simulink model "ScriptDemo"  (R2022b)
settings: configuration reference "TmVcThermal_Configuration_sub" (kept outside this file)
undefined symbols (not defined in the file or in its folder): aaaa, bbbb, cTmComprCtrl_D_u8HvacFlowTable_db, cTmComprCtrl_D_u8HvacFlowTable_sw, cTmComprCtrl_n_i16ChillCmpIMax, cTmComprCtrl_n_i16ChillCmpIMin, cTmComprCtrl_n_i16ChillCmpIMin666, cTmComprCtrl_n_i16ChillCmpPMax, cTmComprCtrl_n_i16ChillCmpPMin, cTmComprCtrl_n_i16CmpChillCoolRpmKiMax, cTmComprCtrl_n_i16CmpChillCoolRpmKiMin, cTmComprCtrl_n_i16CmpChillCoolRpmKpMax, cTmComprCtrl_n_i16CmpChillCoolRpmKpMin, cTmComprCtrl_n_i16CmpCoolRpmKiMax, cTmComprCtrl_n_i16CmpCoolRpmKiMin, cTmComprCtrl_n_i16CmpCoolRpmKpMax, cTmComprCtrl_n_i16CmpCoolRpmKpMin, cTmComprCtrl_n_i16SM4CmpHeatKiMax, cTmComprCtrl_n_i16SM4CmpHeatKiMin, cTmComprCtrl_n_i16SM4CmpHeatKpMax, cTmComprCtrl_n_i16SM4CmpHeatKpMin, cTmComprCtrl_n_i16SM5CmpHeatKiMax, cTmComprCtrl_n_i16SM5CmpHeatKiMin, cTmComprCtrl_n_i16SM5CmpHeatKpMax, cTmComprCtrl_n_i16SM5CmpHeatKpMin, cTmComprCtrl_n_i16SM6CmpHeatKiMax, cTmComprCtrl_n_i16SM6CmpHeatKiMin, cTmComprCtrl_n_i16SM6CmpHeatKpMax, cTmComprCtrl_n_i16SM6CmpHeatKpMin, cTmComprCtrl_n_u16CmpMaxSpdFanFltLimt, cTmComprCtrl_n_u16CmpMaxSpdLoSidePFltLimt, cTmComprCtrl_n_u16CmpMaxSpdSensorFltLimt, cTmComprCtrl_n_u16CompMinRpm, cTmComprCtrl_n_u16CompRpmIncThres, cTmComprCtrl_t_u16BattCooltFFPeriod, cTmComprCtrl_t_u16BattCooltPIPeriod, cTmComprCtrl_t_u16CmpCoolFFPeriod, cTmComprCtrl_t_u16CmpCoolPIPeriod, cTmComprCtrl_t_u16CoolCmpChillFFPeriod, cTmComprCtrl_t_u16CoolCmpChillPIPeriod, cTmComprCtrl_t_u16SM4CmpHeatFFPeriod, cTmComprCtrl_t_u16SM4CmpHeatPIPeriod, cTmComprCtrl_t_u16SM5CmpHeatFFPeriod, cTmComprCtrl_t_u16SM5CmpHeatPIPeriod, cTmComprCtrl_t_u16SM6CmpHeatFFPeriod, cTmComprCtrl_t_u16SM6CmpHeatPIPeriod, cTmComprCtrl_Te_EvapClearInteg, cTmComprCtrl_Te_i16HpReqTempSaturoffset, cTmComprCtrl_Te_i16SatLpReplaceDiff, cTmComprCtrl_Te_i16SM3BatDiffStartEvapDecOffset, cTmComprCtrl_Te_i16SM3EvapLo, cTmComprCtrl_Te_i16SM3TBatDiffEntEvapDecOffset, cTmComprCtrl_Te_i16SM3TBatDiffEntEvapDecOffsetQuit, cTmComprCtrl_Te_s32ErrCmpChillPIContinueCoolH, cTmComprCtrl_Te_s32ErrCmpChillPIContinueCoolL, cTmComprCtrl_Te_s32ErrCmpPIContinueChillH, cTmComprCtrl_Te_s32ErrCmpPIContinueChillL, cTmComprCtrl_Te_s32ErrCmpPIContinueCoolH, cTmComprCtrl_Te_s32ErrCmpPIContinueCoolL, cTmComprCtrl_Te_s32ErrCmpPIContinueHeatH ... (+398)
libraries: simulink x846, PCMULib x711, simulink_need_slupdate x4
(part 18 of 49)

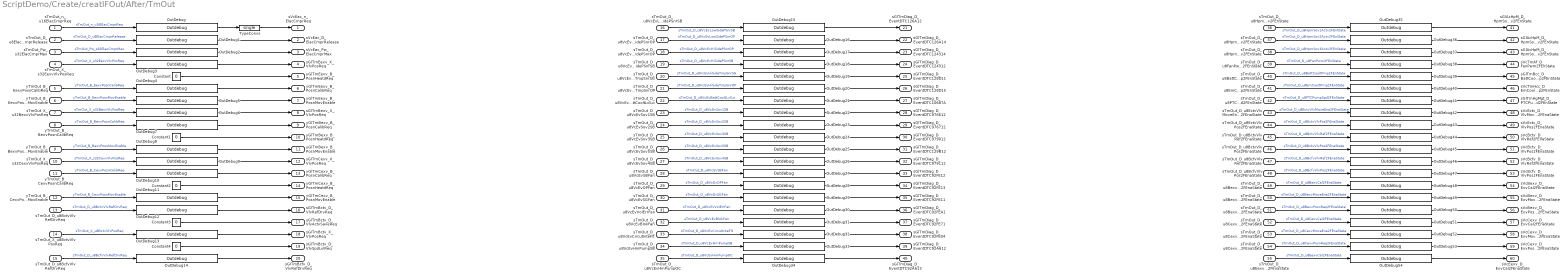
== system ScriptDemo/Create/creatIFOut/After/TmOut ==
  sTmOut_n_u16ElacCmprReq : Inport  OutDataTypeStr=uint16
  sTmOut_D_u8ElacCmprRelease : Inport  Port=2  OutDataTypeStr=uint8
  sTmOut_Pw_s32ElacCmprMax : Inport  Port=3  OutDataTypeStr=single
  sTmOut_X_s32EexvVlvPosReq : Inport  Port=4  OutDataTypeStr=single
  yTmOut_B_EexvPosnCalibReq : Inport  Port=5  OutDataTypeStr=boolean
  yTmOut_B_EexvPosnMovEnable : Inport  Port=6  OutDataTypeStr=boolean
  sTmOut_X_s32BexvVlvPosReq : Inport  Port=7  OutDataTypeStr=single
  yTmOut_B_BexvPosnCalibReq : Inport  Port=8  OutDataTypeStr=boolean
  yTmOut_B_BexvPosnMovEnable : Inport  Port=9  OutDataTypeStr=boolean
  sTmOut_X_s32CexvVlvPosReq : Inport  Port=10  OutDataTypeStr=single
  yTmOut_B_CexvPosnCalibReq : Inport  Port=11  OutDataTypeStr=boolean
  yTmOut_B_CexvPosnMovEnable : Inport  Port=12  OutDataTypeStr=boolean
  sTmOut_D_u8BctvVlvRefDrvReq : Inport  Port=13  OutDataTypeStr=uint8
  sTmOut_X_u8BctvVlvPosReq : Inport  Port=14  OutDataTypeStr=uint8
  sTmOut_D_u8BcfvVlvRefDrvReq : Inport  Port=15  OutDataTypeStr=uint8
  sTmOut_D_u8VcEvLowSidePSnrSB : Inport  Port=16  OutDataTypeStr=uint8
  sTmOut_D_u8VcEvLowSidePSnrOP : Inport  Port=17  OutDataTypeStr=uint8
  sTmOut_D_u8VcEvHiSidePSnrOP : Inport  Port=18  OutDataTypeStr=uint8
  sTmOut_D_u8VcEvHiSidePSnrSB : Inport  Port=19  OutDataTypeStr=uint8
  sTmOut_D_u8VcEvHiSideTmpSnrSG : Inport  Port=20  OutDataTypeStr=uint8
  sTmOut_D_u8VcEvHiSideTmpSnrOP : Inport  Port=21  OutDataTypeStr=uint8
  sTmOut_D_u8VcEvBattCooltLvlLo : Inport  Port=22  OutDataTypeStr=uint8
  sTmOut_D_u8VcEvSov1SB : Inport  Port=23  OutDataTypeStr=uint8
  sTmOut_D_u8VcEvSov2SB : Inport  Port=24  OutDataTypeStr=uint8
  sTmOut_D_u8VcEvSov3SB : Inport  Port=25  OutDataTypeStr=uint8
  sTmOut_D_u8VcEvSov5SB : Inport  Port=26  OutDataTypeStr=uint8
  sTmOut_D_u8VcEvSov4SB : Inport  Port=27  OutDataTypeStr=uint8
  sTmOut_D_u8VcEvSBFan : Inport  Port=28  OutDataTypeStr=uint8
  sTmOut_D_u8VcEvOPFan : Inport  Port=29  OutDataTypeStr=uint8
  sTmOut_D_u8VcEvSGFan : Inport  Port=30  OutDataTypeStr=uint8
  sTmOut_D_u8VcEvVolErrFan : Inport  Port=31  OutDataTypeStr=uint8
  sTmOut_D_u8VcEvBlokFan : Inport  Port=32  OutDataTypeStr=uint8
  sTmOut_D_u8VcEvCircutInteFlt : Inport  Port=33  OutDataTypeStr=uint8
  sTmOut_D_u8VcEvHmPumpSB : Inport  Port=34  OutDataTypeStr=uint8
  sTmOut_D_u8VcEvHmPumpOC : Inport  Port=35  OutDataTypeStr=uint8
  sTmOut_D_u8HpmSov1Actv2FEnState : Inport  Port=36  OutDataTypeStr=uint8
  sTmOut_D_u8HpmSov2Actv2FEnState : Inport  Port=37  OutDataTypeStr=uint8
  sTmOut_D_u8HpmSov3Actv2FEnState : Inport  Port=38  OutDataTypeStr=uint8
  sTmOut_D_u8FanPwm2FEnState : Inport  Port=39  OutDataTypeStr=uint8
  sTmOut_D_u8BattCooltPmp2FEnState : Inport  Port=40  OutDataTypeStr=uint8
  sTmOut_D_u8EmCooltPmp2FEnState : Inport  Port=41  OutDataTypeStr=uint8
  sTmOut_D_u8PTCPumpSpd2FEnState : Inport  Port=42  OutDataTypeStr=uint8
  sTmOut_D_u8EctvVlvMoveEna2FEnaState : Inport  Port=43  OutDataTypeStr=uint8
  sTmOut_D_u8EctvVlvPos2FEnaState : Inport  Port=44  OutDataTypeStr=uint8
  sTmOut_D_u8BctvVlvRef2FEnaState : Inport  Port=45  OutDataTypeStr=uint8
  sTmOut_D_u8BctvVlvPos2FEnaState : Inport  Port=46  OutDataTypeStr=uint8
  sTmOut_D_u8BcfvVlvRef2FEnaState : Inport  Port=47  OutDataTypeStr=uint8
  sTmOut_D_u8BcfvVlvPos2FEnaState : Inport  Port=48  OutDataTypeStr=uint8
  sTmOut_D_u8BexvCal2FEnaState : Inport  Port=49  OutDataTypeStr=uint8
  sTmOut_D_u8BexvMoveEna2FEnaState : Inport  Port=50  OutDataTypeStr=uint8
  sTmOut_D_u8BexvPosnReq2FEnaState : Inport  Port=51  OutDataTypeStr=uint8
  sTmOut_D_u8CexvCal2FEnaState : Inport  Port=52  OutDataTypeStr=uint8
  sTmOut_D_u8CexvMoveEna2FEnaState : Inport  Port=53  OutDataTypeStr=uint8
  sTmOut_D_u8CexvPosnReq2FEnaState : Inport  Port=54  OutDataTypeStr=uint8
  sTmOut_D_u8EexvCal2FEnaState : Inport  Port=55  OutDataTypeStr=uint8
  Constant : Constant  Value=0  OutDataTypeStr=boolean
  Constant1 : Constant  Value=0  OutDataTypeStr=boolean
  Constant2 : Constant  Value=0  OutDataTypeStr=boolean
  Constant3 : Constant  Value=0  OutDataTypeStr=uint8
  Constant4 : Constant  Value=0  OutDataTypeStr=uint8
  OutDebug : PCMULib/Interface/Outdebug  SWI=cTmOut_n_u16ElacCmprReq_sw  DBI=cTmOut_n_u16ElacCmprReq_db
      settings: SourceProductName=PCMULib
  OutDebug1 : PCMULib/Interface/Outdebug  SWI=cTmOut_D_u8ElacCmprRelease_sw  DBI=cTmOut_D_u8ElacCmprRelease_db
      settings: SourceProductName=PCMULib
  OutDebug10 : PCMULib/Interface/Outdebug  SWI=cTmOut_B_CexvPosnCalibReq_sw  DBI=cTmOut_B_CexvPosnCalibReq_db
      settings: SourceProductName=PCMULib
  OutDebug11 : PCMULib/Interface/Outdebug  SWI=cTmOut_B_CexvPosnMovEnable_sw  DBI=cTmOut_B_CexvPosnMovEnable_db
      settings: SourceProductName=PCMULib
  OutDebug12 : PCMULib/Interface/Outdebug  SWI=cTmOut_D_u8BctvVlvRefDrvReq_sw  DBI=cTmOut_D_u8BctvVlvRefDrvReq_db
      settings: SourceProductName=PCMULib
  OutDebug13 : PCMULib/Interface/Outdebug  SWI=cTmOut_X_u8BctvVlvPosReq_sw  DBI=cTmOut_X_u8BctvVlvPosReq_db
      settings: SourceProductName=PCMULib
  OutDebug14 : PCMULib/Interface/Outdebug  SWI=cTmOut_D_u8BcfvVlvRefDrvReq_sw  DBI=cTmOut_D_u8BcfvVlvRefDrvReq_db
      settings: SourceProductName=PCMULib
  OutDebug15 : PCMULib/Interface/Outdebug  SWI=cTmOut_D_u8VcEvLowSidePSnrSB_sw  DBI=cTmOut_D_u8VcEvLowSidePSnrSB_db
      settings: SourceProductName=PCMULib
  OutDebug16 : PCMULib/Interface/Outdebug  SWI=cTmOut_D_u8VcEvLowSidePSnrOP_sw  DBI=cTmOut_D_u8VcEvLowSidePSnrOP_db
      settings: SourceProductName=PCMULib
  OutDebug17 : PCMULib/Interface/Outdebug  SWI=cTmOut_D_u8VcEvHiSidePSnrOP_sw  DBI=cTmOut_D_u8VcEvHiSidePSnrOP_db
      settings: SourceProductName=PCMULib
  OutDebug18 : PCMULib/Interface/Outdebug  SWI=cTmOut_D_u8VcEvHiSidePSnrSB_sw  DBI=cTmOut_D_u8VcEvHiSidePSnrSB_db
      settings: SourceProductName=PCMULib
  OutDebug19 : PCMULib/Interface/Outdebug  SWI=cTmOut_D_u8VcEvHiSideTmpSnrSG_sw  DBI=cTmOut_D_u8VcEvHiSideTmpSnrSG_db
      settings: SourceProductName=PCMULib
  OutDebug2 : PCMULib/Interface/Outdebug  SWI=cTmOut_Pw_s32ElacCmprMax_sw  DBI=cTmOut_Pw_s32ElacCmprMax_db
      settings: SourceProductName=PCMULib
  OutDebug20 : PCMULib/Interface/Outdebug  SWI=cTmOut_D_u8VcEvHiSideTmpSnrOP_sw  DBI=cTmOut_D_u8VcEvHiSideTmpSnrOP_db
      settings: SourceProductName=PCMULib
  OutDebug21 : PCMULib/Interface/Outdebug  SWI=cTmOut_D_u8VcEvBattCooltLvlLo_sw  DBI=cTmOut_D_u8VcEvBattCooltLvlLo_db
      settings: SourceProductName=PCMULib
  OutDebug22 : PCMULib/Interface/Outdebug  SWI=cTmOut_D_u8VcEvSov1SB_sw  DBI=cTmOut_D_u8VcEvSov1SB_db
      settings: SourceProductName=PCMULib
  OutDebug23 : PCMULib/Interface/Outdebug  SWI=cTmOut_D_u8VcEvSov2SB_sw  DBI=cTmOut_D_u8VcEvSov2SB_db
      settings: SourceProductName=PCMULib
  OutDebug24 : PCMULib/Interface/Outdebug  SWI=cTmOut_D_u8VcEvSov3SB_sw  DBI=cTmOut_D_u8VcEvSov3SB_db
      settings: SourceProductName=PCMULib
  OutDebug25 : PCMULib/Interface/Outdebug  SWI=cTmOut_D_u8VcEvSov5SB_sw  DBI=cTmOut_D_u8VcEvSov5SB_db
      settings: SourceProductName=PCMULib
  OutDebug26 : PCMULib/Interface/Outdebug  SWI=cTmOut_D_u8VcEvSov4SB_sw  DBI=cTmOut_D_u8VcEvSov4SB_db
      settings: SourceProductName=PCMULib
  OutDebug27 : PCMULib/Interface/Outdebug  SWI=cTmOut_D_u8VcEvSBFan_sw  DBI=cTmOut_D_u8VcEvSBFan_db
      settings: SourceProductName=PCMULib
  OutDebug28 : PCMULib/Interface/Outdebug  SWI=cTmOut_D_u8VcEvOPFan_sw  DBI=cTmOut_D_u8VcEvOPFan_db
      settings: SourceProductName=PCMULib
  OutDebug29 : PCMULib/Interface/Outdebug  SWI=cTmOut_D_u8VcEvSGFan_sw  DBI=cTmOut_D_u8VcEvSGFan_db
      settings: SourceProductName=PCMULib
  OutDebug3 : PCMULib/Interface/Outdebug  SWI=cTmOut_X_s32EexvVlvPosReq_sw  DBI=cTmOut_X_s32EexvVlvPosReq_db
      settings: SourceProductName=PCMULib
  OutDebug30 : PCMULib/Interface/Outdebug  SWI=cTmOut_D_u8VcEvVolErrFan_sw  DBI=cTmOut_D_u8VcEvVolErrFan_db
      settings: SourceProductName=PCMULib
  OutDebug31 : PCMULib/Interface/Outdebug  SWI=cTmOut_D_u8VcEvBlokFan_sw  DBI=cTmOut_D_u8VcEvBlokFan_db
      settings: SourceProductName=PCMULib
  OutDebug32 : PCMULib/Interface/Outdebug  SWI=cTmOut_D_u8VcEvCircutInteFlt_sw  DBI=cTmOut_D_u8VcEvCircutInteFlt_db
      settings: SourceProductName=PCMULib
  OutDebug33 : PCMULib/Interface/Outdebug  SWI=cTmOut_D_u8VcEvHmPumpSB_sw  DBI=cTmOut_D_u8VcEvHmPumpSB_db
      settings: SourceProductName=PCMULib
  OutDebug34 : PCMULib/Interface/Outdebug  SWI=cTmOut_D_u8VcEvHmPumpOC_sw  DBI=cTmOut_D_u8VcEvHmPumpOC_db
      settings: SourceProductName=PCMULib
  OutDebug35 : PCMULib/Interface/Outdebug  SWI=cTmOut_D_u8HpmSov1Actv2FEnState_sw  DBI=cTmOut_D_u8HpmSov1Actv2FEnState_db
      settings: SourceProductName=PCMULib
  OutDebug36 : PCMULib/Interface/Outdebug  SWI=cTmOut_D_u8HpmSov2Actv2FEnState_sw  DBI=cTmOut_D_u8HpmSov2Actv2FEnState_db
      settings: SourceProductName=PCMULib
  OutDebug37 : PCMULib/Interface/Outdebug  SWI=cTmOut_D_u8HpmSov3Actv2FEnState_sw  DBI=cTmOut_D_u8HpmSov3Actv2FEnState_db
      settings: SourceProductName=PCMULib
  OutDebug38 : PCMULib/Interface/Outdebug  SWI=cTmOut_D_u8FanPwm2FEnState_sw  DBI=cTmOut_D_u8FanPwm2FEnState_db
      settings: SourceProductName=PCMULib
  OutDebug39 : PCMULib/Interface/Outdebug  SWI=cTmOut_D_u8BattCooltPmp2FEnState_sw  DBI=cTmOut_D_u8BattCooltPmp2FEnState_db
      settings: SourceProductName=PCMULib
  OutDebug4 : PCMULib/Interface/Outdebug  SWI=cTmOut_B_EexvPosnCalibReq_sw  DBI=cTmOut_B_EexvPosnCalibReq_db
      settings: SourceProductName=PCMULib
  OutDebug40 : PCMULib/Interface/Outdebug  SWI=cTmOut_D_u8EmCooltPmp2FEnState_sw  DBI=cTmOut_D_u8EmCooltPmp2FEnState_db
      settings: SourceProductName=PCMULib
  OutDebug41 : PCMULib/Interface/Outdebug  SWI=cTmOut_D_u8PTCPumpSpd2FEnState_sw  DBI=cTmOut_D_u8PTCPumpSpd2FEnState_db
      settings: SourceProductName=PCMULib
  OutDebug42 : PCMULib/Interface/Outdebug  SWI=cTmOut_D_u8EctvVlvMoveEna2FEnaState_sw  DBI=cTmOut_D_u8EctvVlvMoveEna2FEnaState_db
      settings: SourceProductName=PCMULib
  OutDebug43 : PCMULib/Interface/Outdebug  SWI=cTmOut_D_u8EctvVlvPos2FEnaState_sw  DBI=cTmOut_D_u8EctvVlvPos2FEnaState_db
      settings: SourceProductName=PCMULib
  OutDebug44 : PCMULib/Interface/Outdebug  SWI=cTmOut_D_u8BctvVlvRef2FEnaState_sw  DBI=cTmOut_D_u8BctvVlvRef2FEnaState_db
      settings: SourceProductName=PCMULib
  OutDebug45 : PCMULib/Interface/Outdebug  SWI=cTmOut_D_u8BctvVlvPos2FEnaState_sw  DBI=cTmOut_D_u8BctvVlvPos2FEnaState_db
      settings: SourceProductName=PCMULib
  OutDebug46 : PCMULib/Interface/Outdebug  SWI=cTmOut_D_u8BcfvVlvRef2FEnaState_sw  DBI=cTmOut_D_u8BcfvVlvRef2FEnaState_db
      settings: SourceProductName=PCMULib
  OutDebug47 : PCMULib/Interface/Outdebug  SWI=cTmOut_D_u8BcfvVlvPos2FEnaState_sw  DBI=cTmOut_D_u8BcfvVlvPos2FEnaState_db
      settings: SourceProductName=PCMULib
  OutDebug48 : PCMULib/Interface/Outdebug  SWI=cTmOut_D_u8BexvCal2FEnaState_sw  DBI=cTmOut_D_u8BexvCal2FEnaState_db
      settings: SourceProductName=PCMULib
  OutDebug49 : PCMULib/Interface/Outdebug  SWI=cTmOut_D_u8BexvMoveEna2FEnaState_sw  DBI=cTmOut_D_u8BexvMoveEna2FEnaState_db
      settings: SourceProductName=PCMULib
  OutDebug5 : PCMULib/Interface/Outdebug  SWI=cTmOut_B_EexvPosnMovEnable_sw  DBI=cTmOut_B_EexvPosnMovEnable_db
      settings: SourceProductName=PCMULib
  OutDebug50 : PCMULib/Interface/Outdebug  SWI=cTmOut_D_u8BexvPosnReq2FEnaState_sw  DBI=cTmOut_D_u8BexvPosnReq2FEnaState_db
      settings: SourceProductName=PCMULib
  OutDebug51 : PCMULib/Interface/Outdebug  SWI=cTmOut_D_u8CexvCal2FEnaState_sw  DBI=cTmOut_D_u8CexvCal2FEnaState_db
      settings: SourceProductName=PCMULib
  OutDebug52 : PCMULib/Interface/Outdebug  SWI=cTmOut_D_u8CexvMoveEna2FEnaState_sw  DBI=cTmOut_D_u8CexvMoveEna2FEnaState_db
      settings: SourceProductName=PCMULib
  OutDebug53 : PCMULib/Interface/Outdebug  SWI=cTmOut_D_u8CexvPosnReq2FEnaState_sw  DBI=cTmOut_D_u8CexvPosnReq2FEnaState_db
      settings: SourceProductName=PCMULib
  OutDebug54 : PCMULib/Interface/Outdebug  SWI=cTmOut_D_u8EexvCal2FEnaState_sw  DBI=cTmOut_D_u8EexvCal2FEnaState_db
      settings: SourceProductName=PCMULib
  OutDebug6 : PCMULib/Interface/Outdebug  SWI=cTmOut_X_s32BexvVlvPosReq_sw  DBI=cTmOut_X_s32BexvVlvPosReq_db
      settings: SourceProductName=PCMULib
  OutDebug7 : PCMULib/Interface/Outdebug  SWI=cTmOut_B_BexvPosnCalibReq_sw  DBI=cTmOut_B_BexvPosnCalibReq_db
      settings: SourceProductName=PCMULib
  OutDebug8 : PCMULib/Interface/Outdebug  SWI=cTmOut_B_BexvPosnMovEnable_sw  DBI=cTmOut_B_BexvPosnMovEnable_db
      settings: SourceProductName=PCMULib
  OutDebug9 : PCMULib/Interface/Outdebug  SWI=cTmOut_X_s32CexvVlvPosReq_sw  DBI=cTmOut_X_s32CexvVlvPosReq_db
      settings: SourceProductName=PCMULib
  TypeConvs : DataTypeConversion  OutDataTypeStr=single
  sVcEac_n_ElacCmprReq : Outport  OutDataTypeStr=single
  sVcEac_D_ElacCmprRelease : Outport  Port=2  OutDataTypeStr=uint8
  sVcEac_Pw_ElacCmprMax : Outport  Port=3  OutDataTypeStr=single
  sGlTmEexv_X_VlvPosReq : Outport  Port=4  OutDataTypeStr=single
  yGlTmEexv_B_PosnHeatdReq : Outport  Port=5  OutDataTypeStr=boolean
  yGlTmEexv_B_PosnCalibReq : Outport  Port=6  OutDataTypeStr=boolean
  yGlTmEexv_B_PosnMovEnable : Outport  Port=7  OutDataTypeStr=boolean
  sGlTmBexv_X_VlvPosReq : Outport  Port=8  OutDataTypeStr=single
  yGlTmBexv_B_PosnCalibReq : Outport  Port=9  OutDataTypeStr=boolean
  yGlTmBexv_B_PosnHeatdReq : Outport  Port=10  OutDataTypeStr=boolean
  yGlTmBexv_B_PosnMovEnable : Outport  Port=11  OutDataTypeStr=boolean
  sGlTmCexv_X_VlvPosReq : Outport  Port=12  OutDataTypeStr=single
  yGlTmCexv_B_PosnCalibReq : Outport  Port=13  OutDataTypeStr=boolean
  yGlTmCexv_B_PosnHeatdReq : Outport  Port=14  OutDataTypeStr=boolean
  yGlTmCexv_B_PosnMovEnable : Outport  Port=15  OutDataTypeStr=boolean
  sGlTmBctv_D_VlvRefDrvReq : Outport  Port=16  OutDataTypeStr=uint8
  sGlTmBctv_D_VlvActvSaveReq : Outport  Port=17  OutDataTypeStr=uint8
  sGlTmBctv_X_VlvPosReq : Outport  Port=18  OutDataTypeStr=uint8
  sGlTmBctv_D_VlvSpdLvlReq : Outport  Port=19  OutDataTypeStr=uint8
  sGlTmBcfv_D_VlvRefDrvReq : Outport  Port=20  OutDataTypeStr=uint8
  sGlTmDiag_D_EventDTC126A12 : Outport  Port=21  OutDataTypeStr=uint8
  sGlTmDiag_D_EventDTC126A14 : Outport  Port=22  OutDataTypeStr=uint8
  sGlTmDiag_D_EventDTC124314 : Outport  Port=23  OutDataTypeStr=uint8
  sGlTmDiag_D_EventDTC124312 : Outport  Port=24  OutDataTypeStr=uint8
  sGlTmDiag_D_EventDTC128D11 : Outport  Port=25  OutDataTypeStr=uint8
  sGlTmDiag_D_EventDTC128D15 : Outport  Port=26  OutDataTypeStr=uint8
  sGlTmDiag_D_EventDTC10687A : Outport  Port=27  OutDataTypeStr=uint8
  sGlTmDiag_D_EventDTC976612 : Outport  Port=28  OutDataTypeStr=uint8
  sGlTmDiag_D_EventDTC976712 : Outport  Port=29  OutDataTypeStr=uint8
  sGlTmDiag_D_EventDTC979012 : Outport  Port=30  OutDataTypeStr=uint8
  sGlTmDiag_D_EventDTC129B12 : Outport  Port=31  OutDataTypeStr=uint8
  sGlTmDiag_D_EventDTC979112 : Outport  Port=32  OutDataTypeStr=uint8
  sGlTmDiag_D_EventDTC92FE12 : Outport  Port=33  OutDataTypeStr=uint8
  sGlTmDiag_D_EventDTC92FE13 : Outport  Port=34  OutDataTypeStr=uint8
  sGlTmDiag_D_EventDTC92FE11 : Outport  Port=35  OutDataTypeStr=uint8
  sGlTmDiag_D_EventDTC92FEA1 : Outport  Port=36  OutDataTypeStr=uint8
  sGlTmDiag_D_EventDTC92FE71 : Outport  Port=37  OutDataTypeStr=uint8
  sGlTmDiag_D_EventDTC92FE04 : Outport  Port=38  OutDataTypeStr=uint8
  sGlTmDiag_D_EventDTC92A612 : Outport  Port=39  OutDataTypeStr=uint8
  sGlTmDiag_D_EventDTC92A613 : Outport  Port=40  OutDataTypeStr=uint8
  sGlAcHpM_D_HpmSov1Actv2FEnState : Outport  Port=41  OutDataTypeStr=uint8
  sGlAcHpM_D_HpmSov2Actv2FEnState : Outport  Port=42  OutDataTypeStr=uint8
  sGlAcHpM_D_HpmSov3Actv2FEnState : Outport  Port=43  OutDataTypeStr=uint8
  sVcTmAf_D_FanPwm2FEnState : Outport  Port=44  OutDataTypeStr=uint8
  sGlTmBcc_D_BattCooltPmp2FEnState : Outport  Port=45  OutDataTypeStr=uint8
  sVcTmHcc_D_EmCooltPmp2FEnState : Outport  Port=46  OutDataTypeStr=uint8
  sGlTmHgMgt_D_PTCPumpSpd2FEnState : Outport  Port=47  OutDataTypeStr=uint8
  sVcEctv_D_VlvMoveEna2FEnaState : Outport  Port=48  OutDataTypeStr=uint8
  sVcEctv_D_VlvPos2FEnaState : Outport  Port=49  OutDataTypeStr=uint8
  sVcBctv_D_VlvRef2FEnaState : Outport  Port=50  OutDataTypeStr=uint8
  sVcBctv_D_VlvPos2FEnaState : Outport  Port=51  OutDataTypeStr=uint8
  sVcBcfv_D_VlvRef2FEnaState : Outport  Port=52  OutDataTypeStr=uint8
  sVcBcfv_D_VlvPos2FEnaState : Outport  Port=53  OutDataTypeStr=uint8
  sVcBexv_D_ExvCal2FEnaState : Outport  Port=54  OutDataTypeStr=uint8
  sVcBexv_D_ExvMoveEna2FEnaState : Outport  Port=55  OutDataTypeStr=uint8
  sVcBexv_D_ExvPosnReq2FEnaState : Outport  Port=56  OutDataTypeStr=uint8
  sVcCexv_D_ExvCal2FEnaState : Outport  Port=57  OutDataTypeStr=uint8
  sVcCexv_D_ExvMoveEna2FEnaState : Outport  Port=58  OutDataTypeStr=uint8
  sVcCexv_D_ExvPosnReq2FEnaState : Outport  Port=59  OutDataTypeStr=uint8
  sVcEexv_D_ExvCal2FEnaState : Outport  Port=60  OutDataTypeStr=uint8
  wires:
  sTmOut_n_u16ElacCmprReq/1 -> OutDebug/1  "sTmOut_n_u16ElacCmprReq"
  OutDebug/1 -> TypeConvs/1
  TypeConvs/1 -> sVcEac_n_ElacCmprReq/1
  sTmOut_D_u8ElacCmprRelease/1 -> OutDebug1/1  "sTmOut_D_u8ElacCmprRelease"
  OutDebug1/1 -> sVcEac_D_ElacCmprRelease/1
  sTmOut_Pw_s32ElacCmprMax/1 -> OutDebug2/1  "sTmOut_Pw_s32ElacCmprMax"
  OutDebug2/1 -> sVcEac_Pw_ElacCmprMax/1
  sTmOut_X_s32EexvVlvPosReq/1 -> OutDebug3/1  "sTmOut_X_s32EexvVlvPosReq"
  OutDebug3/1 -> sGlTmEexv_X_VlvPosReq/1
  Constant/1 -> yGlTmEexv_B_PosnHeatdReq/1
  yTmOut_B_EexvPosnCalibReq/1 -> OutDebug4/1  "yTmOut_B_EexvPosnCalibReq"
  OutDebug4/1 -> yGlTmEexv_B_PosnCalibReq/1
  yTmOut_B_EexvPosnMovEnable/1 -> OutDebug5/1  "yTmOut_B_EexvPosnMovEnable"
  OutDebug5/1 -> yGlTmEexv_B_PosnMovEnable/1
  sTmOut_X_s32BexvVlvPosReq/1 -> OutDebug6/1  "sTmOut_X_s32BexvVlvPosReq"
  OutDebug6/1 -> sGlTmBexv_X_VlvPosReq/1
  yTmOut_B_BexvPosnCalibReq/1 -> OutDebug7/1  "yTmOut_B_BexvPosnCalibReq"
  OutDebug7/1 -> yGlTmBexv_B_PosnCalibReq/1
  Constant1/1 -> yGlTmBexv_B_PosnHeatdReq/1
  yTmOut_B_BexvPosnMovEnable/1 -> OutDebug8/1  "yTmOut_B_BexvPosnMovEnable"
  OutDebug8/1 -> yGlTmBexv_B_PosnMovEnable/1
  sTmOut_X_s32CexvVlvPosReq/1 -> OutDebug9/1  "sTmOut_X_s32CexvVlvPosReq"
  OutDebug9/1 -> sGlTmCexv_X_VlvPosReq/1
  yTmOut_B_CexvPosnCalibReq/1 -> OutDebug10/1  "yTmOut_B_CexvPosnCalibReq"
  OutDebug10/1 -> yGlTmCexv_B_PosnCalibReq/1
  Constant2/1 -> yGlTmCexv_B_PosnHeatdReq/1
  yTmOut_B_CexvPosnMovEnable/1 -> OutDebug11/1  "yTmOut_B_CexvPosnMovEnable"
  OutDebug11/1 -> yGlTmCexv_B_PosnMovEnable/1
  sTmOut_D_u8BctvVlvRefDrvReq/1 -> OutDebug12/1  "sTmOut_D_u8BctvVlvRefDrvReq"
  OutDebug12/1 -> sGlTmBctv_D_VlvRefDrvReq/1
  Constant3/1 -> sGlTmBctv_D_VlvActvSaveReq/1
  sTmOut_X_u8BctvVlvPosReq/1 -> OutDebug13/1  "sTmOut_X_u8BctvVlvPosReq"
  OutDebug13/1 -> sGlTmBctv_X_VlvPosReq/1
  Constant4/1 -> sGlTmBctv_D_VlvSpdLvlReq/1
  sTmOut_D_u8BcfvVlvRefDrvReq/1 -> OutDebug14/1  "sTmOut_D_u8BcfvVlvRefDrvReq"
  OutDebug14/1 -> sGlTmBcfv_D_VlvRefDrvReq/1
  sTmOut_D_u8VcEvLowSidePSnrSB/1 -> OutDebug15/1  "sTmOut_D_u8VcEvLowSidePSnrSB"
  OutDebug15/1 -> sGlTmDiag_D_EventDTC126A12/1
  sTmOut_D_u8VcEvLowSidePSnrOP/1 -> OutDebug16/1  "sTmOut_D_u8VcEvLowSidePSnrOP"
  OutDebug16/1 -> sGlTmDiag_D_EventDTC126A14/1
  sTmOut_D_u8VcEvHiSidePSnrOP/1 -> OutDebug17/1  "sTmOut_D_u8VcEvHiSidePSnrOP"
  OutDebug17/1 -> sGlTmDiag_D_EventDTC124314/1
  sTmOut_D_u8VcEvHiSidePSnrSB/1 -> OutDebug18/1  "sTmOut_D_u8VcEvHiSidePSnrSB"
  OutDebug18/1 -> sGlTmDiag_D_EventDTC124312/1
  sTmOut_D_u8VcEvHiSideTmpSnrSG/1 -> OutDebug19/1  "sTmOut_D_u8VcEvHiSideTmpSnrSG"
  OutDebug19/1 -> sGlTmDiag_D_EventDTC128D11/1
  sTmOut_D_u8VcEvHiSideTmpSnrOP/1 -> OutDebug20/1  "sTmOut_D_u8VcEvHiSideTmpSnrOP"
  OutDebug20/1 -> sGlTmDiag_D_EventDTC128D15/1
  sTmOut_D_u8VcEvBattCooltLvlLo/1 -> OutDebug21/1  "sTmOut_D_u8VcEvBattCooltLvlLo"
  OutDebug21/1 -> sGlTmDiag_D_EventDTC10687A/1
  sTmOut_D_u8VcEvSov1SB/1 -> OutDebug22/1  "sTmOut_D_u8VcEvSov1SB"
  OutDebug22/1 -> sGlTmDiag_D_EventDTC976612/1
  sTmOut_D_u8VcEvSov2SB/1 -> OutDebug23/1  "sTmOut_D_u8VcEvSov2SB"
  OutDebug23/1 -> sGlTmDiag_D_EventDTC976712/1
  sTmOut_D_u8VcEvSov3SB/1 -> OutDebug24/1  "sTmOut_D_u8VcEvSov3SB"
  OutDebug24/1 -> sGlTmDiag_D_EventDTC979012/1
  sTmOut_D_u8VcEvSov5SB/1 -> OutDebug25/1  "sTmOut_D_u8VcEvSov5SB"
  OutDebug25/1 -> sGlTmDiag_D_EventDTC129B12/1
  sTmOut_D_u8VcEvSov4SB/1 -> OutDebug26/1  "sTmOut_D_u8VcEvSov4SB"
  OutDebug26/1 -> sGlTmDiag_D_EventDTC979112/1
  sTmOut_D_u8VcEvSBFan/1 -> OutDebug27/1  "sTmOut_D_u8VcEvSBFan"
  OutDebug27/1 -> sGlTmDiag_D_EventDTC92FE12/1
  sTmOut_D_u8VcEvOPFan/1 -> OutDebug28/1  "sTmOut_D_u8VcEvOPFan"
  OutDebug28/1 -> sGlTmDiag_D_EventDTC92FE13/1
  sTmOut_D_u8VcEvSGFan/1 -> OutDebug29/1  "sTmOut_D_u8VcEvSGFan"
  OutDebug29/1 -> sGlTmDiag_D_EventDTC92FE11/1
  sTmOut_D_u8VcEvVolErrFan/1 -> OutDebug30/1  "sTmOut_D_u8VcEvVolErrFan"
  OutDebug30/1 -> sGlTmDiag_D_EventDTC92FEA1/1
  sTmOut_D_u8VcEvBlokFan/1 -> OutDebug31/1  "sTmOut_D_u8VcEvBlokFan"
  OutDebug31/1 -> sGlTmDiag_D_EventDTC92FE71/1
  sTmOut_D_u8VcEvCircutInteFlt/1 -> OutDebug32/1  "sTmOut_D_u8VcEvCircutInteFlt"
  OutDebug32/1 -> sGlTmDiag_D_EventDTC92FE04/1
  sTmOut_D_u8VcEvHmPumpSB/1 -> OutDebug33/1  "sTmOut_D_u8VcEvHmPumpSB"
  OutDebug33/1 -> sGlTmDiag_D_EventDTC92A612/1
  sTmOut_D_u8VcEvHmPumpOC/1 -> OutDebug34/1  "sTmOut_D_u8VcEvHmPumpOC"
  OutDebug34/1 -> sGlTmDiag_D_EventDTC92A613/1
  sTmOut_D_u8HpmSov1Actv2FEnState/1 -> OutDebug35/1  "sTmOut_D_u8HpmSov1Actv2FEnState"
  OutDebug35/1 -> sGlAcHpM_D_HpmSov1Actv2FEnState/1
  sTmOut_D_u8HpmSov2Actv2FEnState/1 -> OutDebug36/1  "sTmOut_D_u8HpmSov2Actv2FEnState"
  OutDebug36/1 -> sGlAcHpM_D_HpmSov2Actv2FEnState/1
  sTmOut_D_u8HpmSov3Actv2FEnState/1 -> OutDebug37/1  "sTmOut_D_u8HpmSov3Actv2FEnState"
  OutDebug37/1 -> sGlAcHpM_D_HpmSov3Actv2FEnState/1
  sTmOut_D_u8FanPwm2FEnState/1 -> OutDebug38/1  "sTmOut_D_u8FanPwm2FEnState"
  OutDebug38/1 -> sVcTmAf_D_FanPwm2FEnState/1
  sTmOut_D_u8BattCooltPmp2FEnState/1 -> OutDebug39/1  "sTmOut_D_u8BattCooltPmp2FEnState"
  OutDebug39/1 -> sGlTmBcc_D_BattCooltPmp2FEnState/1
  sTmOut_D_u8EmCooltPmp2FEnState/1 -> OutDebug40/1  "sTmOut_D_u8EmCooltPmp2FEnState"
  OutDebug40/1 -> sVcTmHcc_D_EmCooltPmp2FEnState/1
  sTmOut_D_u8PTCPumpSpd2FEnState/1 -> OutDebug41/1  "sTmOut_D_u8PTCPumpSpd2FEnState"
  OutDebug41/1 -> sGlTmHgMgt_D_PTCPumpSpd2FEnState/1
  sTmOut_D_u8EctvVlvMoveEna2FEnaState/1 -> OutDebug42/1  "sTmOut_D_u8EctvVlvMoveEna2FEnaState"
  OutDebug42/1 -> sVcEctv_D_VlvMoveEna2FEnaState/1
  sTmOut_D_u8EctvVlvPos2FEnaState/1 -> OutDebug43/1  "sTmOut_D_u8EctvVlvPos2FEnaState"
  OutDebug43/1 -> sVcEctv_D_VlvPos2FEnaState/1
  sTmOut_D_u8BctvVlvRef2FEnaState/1 -> OutDebug44/1  "sTmOut_D_u8BctvVlvRef2FEnaState"
  OutDebug44/1 -> sVcBctv_D_VlvRef2FEnaState/1
  sTmOut_D_u8BctvVlvPos2FEnaState/1 -> OutDebug45/1  "sTmOut_D_u8BctvVlvPos2FEnaState"
  OutDebug45/1 -> sVcBctv_D_VlvPos2FEnaState/1
  sTmOut_D_u8BcfvVlvRef2FEnaState/1 -> OutDebug46/1  "sTmOut_D_u8BcfvVlvRef2FEnaState"
  OutDebug46/1 -> sVcBcfv_D_VlvRef2FEnaState/1
  sTmOut_D_u8BcfvVlvPos2FEnaState/1 -> OutDebug47/1  "sTmOut_D_u8BcfvVlvPos2FEnaState"
  OutDebug47/1 -> sVcBcfv_D_VlvPos2FEnaState/1
  sTmOut_D_u8BexvCal2FEnaState/1 -> OutDebug48/1  "sTmOut_D_u8BexvCal2FEnaState"
  OutDebug48/1 -> sVcBexv_D_ExvCal2FEnaState/1
  sTmOut_D_u8BexvMoveEna2FEnaState/1 -> OutDebug49/1  "sTmOut_D_u8BexvMoveEna2FEnaState"
  OutDebug49/1 -> sVcBexv_D_ExvMoveEna2FEnaState/1
  sTmOut_D_u8BexvPosnReq2FEnaState/1 -> OutDebug50/1  "sTmOut_D_u8BexvPosnReq2FEnaState"
  OutDebug50/1 -> sVcBexv_D_ExvPosnReq2FEnaState/1
  sTmOut_D_u8CexvCal2FEnaState/1 -> OutDebug51/1  "sTmOut_D_u8CexvCal2FEnaState"
  OutDebug51/1 -> sVcCexv_D_ExvCal2FEnaState/1
  sTmOut_D_u8CexvMoveEna2FEnaState/1 -> OutDebug52/1  "sTmOut_D_u8CexvMoveEna2FEnaState"
  OutDebug52/1 -> sVcCexv_D_ExvMoveEna2FEnaState/1
  sTmOut_D_u8CexvPosnReq2FEnaState/1 -> OutDebug53/1  "sTmOut_D_u8CexvPosnReq2FEnaState"
  OutDebug53/1 -> sVcCexv_D_ExvPosnReq2FEnaState/1
  sTmOut_D_u8EexvCal2FEnaState/1 -> OutDebug54/1  "sTmOut_D_u8EexvCal2FEnaState"
  OutDebug54/1 -> sVcEexv_D_ExvCal2FEnaState/1

== system ScriptDemo/Create/creatTmOut/Before/TmBase2Out ==
  sTmComprCtrl_n_u16CompRpmReq : Inport  OutDataTypeStr=uint16
  yTmComprCtrl_B_CompOnReq : Inport  Port=2  OutDataTypeStr=boolean
  sTmEnergyMgr_Pw_s32AcCmprPwrLim : Inport  Port=3  OutDataTypeStr=single
  sTmRefriVlvCtrl_X_s32EEXVPosReq : Inport  Port=4  OutDataTypeStr=single
  yTmRefriVlvCtrl_B_EexvCalibReq : Inport  Port=5  OutDataTypeStr=boolean
  yTmRefriVlvCtrl_B_HpcEexvMovEnable : Inport  Port=6  OutDataTypeStr=boolean
  sTmRefriVlvCtrl_X_s32BEXVPosReq : Inport  Port=7  OutDataTypeStr=single
  yTmRefriVlvCtrl_B_BexvCalibReq : Inport  Port=8  OutDataTypeStr=boolean
  yTmRefriVlvCtrl_B_HpcBexvMovEnable : Inport  Port=9  OutDataTypeStr=boolean
  sTmRefriVlvCtrl_X_s32CEXVPosReq : Inport  Port=10  OutDataTypeStr=single
  yTmRefriVlvCtrl_B_CexvCalibReq : Inport  Port=11  OutDataTypeStr=boolean
  yTmRefriVlvCtrl_B_HpcCexvMovEnable : Inport  Port=12  OutDataTypeStr=boolean
  sTmColtVlvCtrl_D_u8HpcBctvRefDrvReq : Inport  Port=13  OutDataTypeStr=uint8
  sTmColtVlvCtrl_X_u8BctvPosReq : Inport  Port=14  OutDataTypeStr=uint8
  sTmColtVlvCtrl_D_u8HpcBcfvRefDrvReq : Inport  Port=15  OutDataTypeStr=uint8
  sTmDiag_D_u8VcEvLowSidePSnrSB : Inport  Port=16  OutDataTypeStr=uint8
  sTmDiag_D_u8VcEvLowSidePSnrOP : Inport  Port=17  OutDataTypeStr=uint8
  sTmDiag_D_u8VcEvHiSidePSnrOP : Inport  Port=18  OutDataTypeStr=uint8
  sTmDiag_D_u8VcEvHiSidePSnrSB : Inport  Port=19  OutDataTypeStr=uint8
  sTmDiag_D_u8VcEvHiSideTmpSnrSG : Inport  Port=20  OutDataTypeStr=uint8
  sTmDiag_D_u8VcEvHiSideTmpSnrOP : Inport  Port=21  OutDataTypeStr=uint8
  sTmDiag_D_u8VcEvBattCooltLvlLo : Inport  Port=22  OutDataTypeStr=uint8
  sTmDiag_D_u8VcEvSov1SB : Inport  Port=23  OutDataTypeStr=uint8
  sTmDiag_D_u8VcEvSov2SB : Inport  Port=24  OutDataTypeStr=uint8
  sTmDiag_D_u8VcEvSov3SB : Inport  Port=25  OutDataTypeStr=uint8
  sTmDiag_D_u8VcEvSov5SB : Inport  Port=26  OutDataTypeStr=uint8
  sTmDiag_D_u8VcEvSov4SB : Inport  Port=27  OutDataTypeStr=uint8
  sTmDiag_D_u8VcEvSBFan : Inport  Port=28  OutDataTypeStr=uint8
  sTmDiag_D_u8VcEvOPFan : Inport  Port=29  OutDataTypeStr=uint8
  sTmDiag_D_u8VcEvSGFan : Inport  Port=30  OutDataTypeStr=uint8
  sTmDiag_D_u8VcEvVolErrFan : Inport  Port=31  OutDataTypeStr=uint8
  sTmDiag_D_u8VcEvBlokFan : Inport  Port=32  OutDataTypeStr=uint8
  sTmDiag_D_u8VcEvCircutInteFlt : Inport  Port=33  OutDataTypeStr=uint8
  sTmDiag_D_u8VcEvHmPumpSB : Inport  Port=34  OutDataTypeStr=uint8
  sTmDiag_D_u8VcEvHmPumpOC : Inport  Port=35  OutDataTypeStr=uint8
  sTmDiag_D_u8HpmSov1Actv2FEnState : Inport  Port=36  OutDataTypeStr=uint8
  sTmDiag_D_u8HpmSov2Actv2FEnState : Inport  Port=37  OutDataTypeStr=uint8
  sTmDiag_D_u8HpmSov3Actv2FEnState : Inport  Port=38  OutDataTypeStr=uint8
  sTmDiag_D_u8FanPwm2FEnState : Inport  Port=39  OutDataTypeStr=uint8
  sTmDiag_D_u8BattCooltPmp2FEnState : Inport  Port=40  OutDataTypeStr=uint8
  sTmDiag_D_u8EmCooltPmp2FEnState : Inport  Port=41  OutDataTypeStr=uint8
  sTmDiag_D_u8PTCPumpSpd2FEnState : Inport  Port=42  OutDataTypeStr=uint8
  sTmDiag_D_u8EctvVlvMoveEna2FEnaState : Inport  Port=43  OutDataTypeStr=uint8
  sTmDiag_D_u8EctvVlvPos2FEnaState : Inport  Port=44  OutDataTypeStr=uint8
  sTmDiag_D_u8BctvVlvRef2FEnaState : Inport  Port=45  OutDataTypeStr=uint8
  sTmDiag_D_u8BctvVlvPos2FEnaState : Inport  Port=46  OutDataTypeStr=uint8
  sTmDiag_D_u8BcfvVlvRef2FEnaState : Inport  Port=47  OutDataTypeStr=uint8
  sTmDiag_D_u8BcfvVlvPos2FEnaState : Inport  Port=48  OutDataTypeStr=uint8
  sTmDiag_D_u8BexvCal2FEnaState : Inport  Port=49  OutDataTypeStr=uint8
  sTmDiag_D_u8BexvMoveEna2FEnaState : Inport  Port=50  OutDataTypeStr=uint8
  sTmDiag_D_u8BexvPosnReq2FEnaState : Inport  Port=51  OutDataTypeStr=uint8
  sTmDiag_D_u8CexvCal2FEnaState : Inport  Port=52  OutDataTypeStr=uint8
  sTmDiag_D_u8CexvMoveEna2FEnaState : Inport  Port=53  OutDataTypeStr=uint8
  sTmDiag_D_u8CexvPosnReq2FEnaState : Inport  Port=54  OutDataTypeStr=uint8
  sTmDiag_D_u8EexvCal2FEnaState : Inport  Port=55  OutDataTypeStr=uint8
  Conversion{,1..54} (55 alike) : SignalConversion  OverrideOpt=off
  TypeConvs : DataTypeConversion  OutDataTypeStr=uint8
  sTmOut_n_u16ElacCmprReq : Outport  OutDataTypeStr=uint16
  sTmOut_D_u8ElacCmprRelease : Outport  Port=2  OutDataTypeStr=uint8
  sTmOut_Pw_s32ElacCmprMax : Outport  Port=3  OutDataTypeStr=single
  sTmOut_X_s32EexvVlvPosReq : Outport  Port=4  OutDataTypeStr=single
  yTmOut_B_EexvPosnCalibReq : Outport  Port=5  OutDataTypeStr=boolean
  yTmOut_B_EexvPosnMovEnable : Outport  Port=6  OutDataTypeStr=boolean
  sTmOut_X_s32BexvVlvPosReq : Outport  Port=7  OutDataTypeStr=single
  yTmOut_B_BexvPosnCalibReq : Outport  Port=8  OutDataTypeStr=boolean
  yTmOut_B_BexvPosnMovEnable : Outport  Port=9  OutDataTypeStr=boolean
  sTmOut_X_s32CexvVlvPosReq : Outport  Port=10  OutDataTypeStr=single
  yTmOut_B_CexvPosnCalibReq : Outport  Port=11  OutDataTypeStr=boolean
  yTmOut_B_CexvPosnMovEnable : Outport  Port=12  OutDataTypeStr=boolean
  sTmOut_D_u8BctvVlvRefDrvReq : Outport  Port=13  OutDataTypeStr=uint8
  sTmOut_X_u8BctvVlvPosReq : Outport  Port=14  OutDataTypeStr=uint8
  sTmOut_D_u8BcfvVlvRefDrvReq : Outport  Port=15  OutDataTypeStr=uint8
  sTmOut_D_u8VcEvLowSidePSnrSB : Outport  Port=16  OutDataTypeStr=uint8
  sTmOut_D_u8VcEvLowSidePSnrOP : Outport  Port=17  OutDataTypeStr=uint8
  sTmOut_D_u8VcEvHiSidePSnrOP : Outport  Port=18  OutDataTypeStr=uint8
  sTmOut_D_u8VcEvHiSidePSnrSB : Outport  Port=19  OutDataTypeStr=uint8
  sTmOut_D_u8VcEvHiSideTmpSnrSG : Outport  Port=20  OutDataTypeStr=uint8
  sTmOut_D_u8VcEvHiSideTmpSnrOP : Outport  Port=21  OutDataTypeStr=uint8
  sTmOut_D_u8VcEvBattCooltLvlLo : Outport  Port=22  OutDataTypeStr=uint8
  sTmOut_D_u8VcEvSov1SB : Outport  Port=23  OutDataTypeStr=uint8
  sTmOut_D_u8VcEvSov2SB : Outport  Port=24  OutDataTypeStr=uint8
  sTmOut_D_u8VcEvSov3SB : Outport  Port=25  OutDataTypeStr=uint8
  sTmOut_D_u8VcEvSov5SB : Outport  Port=26  OutDataTypeStr=uint8
  sTmOut_D_u8VcEvSov4SB : Outport  Port=27  OutDataTypeStr=uint8
  sTmOut_D_u8VcEvSBFan : Outport  Port=28  OutDataTypeStr=uint8
  sTmOut_D_u8VcEvOPFan : Outport  Port=29  OutDataTypeStr=uint8
  sTmOut_D_u8VcEvSGFan : Outport  Port=30  OutDataTypeStr=uint8
  sTmOut_D_u8VcEvVolErrFan : Outport  Port=31  OutDataTypeStr=uint8
  sTmOut_D_u8VcEvBlokFan : Outport  Port=32  OutDataTypeStr=uint8
  sTmOut_D_u8VcEvCircutInteFlt : Outport  Port=33  OutDataTypeStr=uint8
  sTmOut_D_u8VcEvHmPumpSB : Outport  Port=34  OutDataTypeStr=uint8
  sTmOut_D_u8VcEvHmPumpOC : Outport  Port=35  OutDataTypeStr=uint8
  sTmOut_D_u8HpmSov1Actv2FEnState : Outport  Port=36  OutDataTypeStr=uint8
  sTmOut_D_u8HpmSov2Actv2FEnState : Outport  Port=37  OutDataTypeStr=uint8
  sTmOut_D_u8HpmSov3Actv2FEnState : Outport  Port=38  OutDataTypeStr=uint8
  sTmOut_D_u8FanPwm2FEnState : Outport  Port=39  OutDataTypeStr=uint8
  sTmOut_D_u8BattCooltPmp2FEnState : Outport  Port=40  OutDataTypeStr=uint8
  sTmOut_D_u8EmCooltPmp2FEnState : Outport  Port=41  OutDataTypeStr=uint8
  sTmOut_D_u8PTCPumpSpd2FEnState : Outport  Port=42  OutDataTypeStr=uint8
  sTmOut_D_u8EctvVlvMoveEna2FEnaState : Outport  Port=43  OutDataTypeStr=uint8
  sTmOut_D_u8EctvVlvPos2FEnaState : Outport  Port=44  OutDataTypeStr=uint8
  sTmOut_D_u8BctvVlvRef2FEnaState : Outport  Port=45  OutDataTypeStr=uint8
  sTmOut_D_u8BctvVlvPos2FEnaState : Outport  Port=46  OutDataTypeStr=uint8
  sTmOut_D_u8BcfvVlvRef2FEnaState : Outport  Port=47  OutDataTypeStr=uint8
  sTmOut_D_u8BcfvVlvPos2FEnaState : Outport  Port=48  OutDataTypeStr=uint8
  sTmOut_D_u8BexvCal2FEnaState : Outport  Port=49  OutDataTypeStr=uint8
  sTmOut_D_u8BexvMoveEna2FEnaState : Outport  Port=50  OutDataTypeStr=uint8
  sTmOut_D_u8BexvPosnReq2FEnaState : Outport  Port=51  OutDataTypeStr=uint8
  sTmOut_D_u8CexvCal2FEnaState : Outport  Port=52  OutDataTypeStr=uint8
  sTmOut_D_u8CexvMoveEna2FEnaState : Outport  Port=53  OutDataTypeStr=uint8
  sTmOut_D_u8CexvPosnReq2FEnaState : Outport  Port=54  OutDataTypeStr=uint8
  sTmOut_D_u8EexvCal2FEnaState : Outport  Port=55  OutDataTypeStr=uint8
  wires:
  sTmComprCtrl_n_u16CompRpmReq/1 -> Conversion/1
  Conversion/1 -> sTmOut_n_u16ElacCmprReq/1  "sTmOut_n_u16ElacCmprReq"
  yTmComprCtrl_B_CompOnReq/1 -> Conversion1/1
  Conversion1/1 -> TypeConvs/1
  TypeConvs/1 -> sTmOut_D_u8ElacCmprRelease/1  "sTmOut_D_u8ElacCmprRelease"
  sTmEnergyMgr_Pw_s32AcCmprPwrLim/1 -> Conversion2/1
  Conversion2/1 -> sTmOut_Pw_s32ElacCmprMax/1  "sTmOut_Pw_s32ElacCmprMax"
  sTmRefriVlvCtrl_X_s32EEXVPosReq/1 -> Conversion3/1
  Conversion3/1 -> sTmOut_X_s32EexvVlvPosReq/1  "sTmOut_X_s32EexvVlvPosReq"
  yTmRefriVlvCtrl_B_EexvCalibReq/1 -> Conversion4/1
  Conversion4/1 -> yTmOut_B_EexvPosnCalibReq/1  "yTmOut_B_EexvPosnCalibReq"
  yTmRefriVlvCtrl_B_HpcEexvMovEnable/1 -> Conversion5/1
  Conversion5/1 -> yTmOut_B_EexvPosnMovEnable/1  "yTmOut_B_EexvPosnMovEnable"
  sTmRefriVlvCtrl_X_s32BEXVPosReq/1 -> Conversion6/1
  Conversion6/1 -> sTmOut_X_s32BexvVlvPosReq/1  "sTmOut_X_s32BexvVlvPosReq"
  yTmRefriVlvCtrl_B_BexvCalibReq/1 -> Conversion7/1
  Conversion7/1 -> yTmOut_B_BexvPosnCalibReq/1  "yTmOut_B_BexvPosnCalibReq"
  yTmRefriVlvCtrl_B_HpcBexvMovEnable/1 -> Conversion8/1
  Conversion8/1 -> yTmOut_B_BexvPosnMovEnable/1  "yTmOut_B_BexvPosnMovEnable"
  sTmRefriVlvCtrl_X_s32CEXVPosReq/1 -> Conversion9/1
  Conversion9/1 -> sTmOut_X_s32CexvVlvPosReq/1  "sTmOut_X_s32CexvVlvPosReq"
  yTmRefriVlvCtrl_B_CexvCalibReq/1 -> Conversion10/1
  Conversion10/1 -> yTmOut_B_CexvPosnCalibReq/1  "yTmOut_B_CexvPosnCalibReq"
  yTmRefriVlvCtrl_B_HpcCexvMovEnable/1 -> Conversion11/1
  Conversion11/1 -> yTmOut_B_CexvPosnMovEnable/1  "yTmOut_B_CexvPosnMovEnable"
  sTmColtVlvCtrl_D_u8HpcBctvRefDrvReq/1 -> Conversion12/1
  Conversion12/1 -> sTmOut_D_u8BctvVlvRefDrvReq/1  "sTmOut_D_u8BctvVlvRefDrvReq"
  sTmColtVlvCtrl_X_u8BctvPosReq/1 -> Conversion13/1
  Conversion13/1 -> sTmOut_X_u8BctvVlvPosReq/1  "sTmOut_X_u8BctvVlvPosReq"
  sTmColtVlvCtrl_D_u8HpcBcfvRefDrvReq/1 -> Conversion14/1
  Conversion14/1 -> sTmOut_D_u8BcfvVlvRefDrvReq/1  "sTmOut_D_u8BcfvVlvRefDrvReq"
  sTmDiag_D_u8VcEvLowSidePSnrSB/1 -> Conversion15/1
  Conversion15/1 -> sTmOut_D_u8VcEvLowSidePSnrSB/1  "sTmOut_D_u8VcEvLowSidePSnrSB"
  sTmDiag_D_u8VcEvLowSidePSnrOP/1 -> Conversion16/1
  Conversion16/1 -> sTmOut_D_u8VcEvLowSidePSnrOP/1  "sTmOut_D_u8VcEvLowSidePSnrOP"
  sTmDiag_D_u8VcEvHiSidePSnrOP/1 -> Conversion17/1
  Conversion17/1 -> sTmOut_D_u8VcEvHiSidePSnrOP/1  "sTmOut_D_u8VcEvHiSidePSnrOP"
  sTmDiag_D_u8VcEvHiSidePSnrSB/1 -> Conversion18/1
  Conversion18/1 -> sTmOut_D_u8VcEvHiSidePSnrSB/1  "sTmOut_D_u8VcEvHiSidePSnrSB"
  sTmDiag_D_u8VcEvHiSideTmpSnrSG/1 -> Conversion19/1
  Conversion19/1 -> sTmOut_D_u8VcEvHiSideTmpSnrSG/1  "sTmOut_D_u8VcEvHiSideTmpSnrSG"
  sTmDiag_D_u8VcEvHiSideTmpSnrOP/1 -> Conversion20/1
  Conversion20/1 -> sTmOut_D_u8VcEvHiSideTmpSnrOP/1  "sTmOut_D_u8VcEvHiSideTmpSnrOP"
  sTmDiag_D_u8VcEvBattCooltLvlLo/1 -> Conversion21/1
  Conversion21/1 -> sTmOut_D_u8VcEvBattCooltLvlLo/1  "sTmOut_D_u8VcEvBattCooltLvlLo"
  sTmDiag_D_u8VcEvSov1SB/1 -> Conversion22/1
  Conversion22/1 -> sTmOut_D_u8VcEvSov1SB/1  "sTmOut_D_u8VcEvSov1SB"
  sTmDiag_D_u8VcEvSov2SB/1 -> Conversion23/1
  Conversion23/1 -> sTmOut_D_u8VcEvSov2SB/1  "sTmOut_D_u8VcEvSov2SB"
  sTmDiag_D_u8VcEvSov3SB/1 -> Conversion24/1
  Conversion24/1 -> sTmOut_D_u8VcEvSov3SB/1  "sTmOut_D_u8VcEvSov3SB"
  sTmDiag_D_u8VcEvSov5SB/1 -> Conversion25/1
  Conversion25/1 -> sTmOut_D_u8VcEvSov5SB/1  "sTmOut_D_u8VcEvSov5SB"
  sTmDiag_D_u8VcEvSov4SB/1 -> Conversion26/1
  Conversion26/1 -> sTmOut_D_u8VcEvSov4SB/1  "sTmOut_D_u8VcEvSov4SB"
  sTmDiag_D_u8VcEvSBFan/1 -> Conversion27/1
  Conversion27/1 -> sTmOut_D_u8VcEvSBFan/1  "sTmOut_D_u8VcEvSBFan"
  sTmDiag_D_u8VcEvOPFan/1 -> Conversion28/1
  Conversion28/1 -> sTmOut_D_u8VcEvOPFan/1  "sTmOut_D_u8VcEvOPFan"
  sTmDiag_D_u8VcEvSGFan/1 -> Conversion29/1
  Conversion29/1 -> sTmOut_D_u8VcEvSGFan/1  "sTmOut_D_u8VcEvSGFan"
  sTmDiag_D_u8VcEvVolErrFan/1 -> Conversion30/1
  Conversion30/1 -> sTmOut_D_u8VcEvVolErrFan/1  "sTmOut_D_u8VcEvVolErrFan"
  sTmDiag_D_u8VcEvBlokFan/1 -> Conversion31/1
  Conversion31/1 -> sTmOut_D_u8VcEvBlokFan/1  "sTmOut_D_u8VcEvBlokFan"
  sTmDiag_D_u8VcEvCircutInteFlt/1 -> Conversion32/1
  Conversion32/1 -> sTmOut_D_u8VcEvCircutInteFlt/1  "sTmOut_D_u8VcEvCircutInteFlt"
  sTmDiag_D_u8VcEvHmPumpSB/1 -> Conversion33/1
  Conversion33/1 -> sTmOut_D_u8VcEvHmPumpSB/1  "sTmOut_D_u8VcEvHmPumpSB"
  sTmDiag_D_u8VcEvHmPumpOC/1 -> Conversion34/1
  Conversion34/1 -> sTmOut_D_u8VcEvHmPumpOC/1  "sTmOut_D_u8VcEvHmPumpOC"
  sTmDiag_D_u8HpmSov1Actv2FEnState/1 -> Conversion35/1
  Conversion35/1 -> sTmOut_D_u8HpmSov1Actv2FEnState/1  "sTmOut_D_u8HpmSov1Actv2FEnState"
  sTmDiag_D_u8HpmSov2Actv2FEnState/1 -> Conversion36/1
  Conversion36/1 -> sTmOut_D_u8HpmSov2Actv2FEnState/1  "sTmOut_D_u8HpmSov2Actv2FEnState"
  sTmDiag_D_u8HpmSov3Actv2FEnState/1 -> Conversion37/1
  Conversion37/1 -> sTmOut_D_u8HpmSov3Actv2FEnState/1  "sTmOut_D_u8HpmSov3Actv2FEnState"
  sTmDiag_D_u8FanPwm2FEnState/1 -> Conversion38/1
  Conversion38/1 -> sTmOut_D_u8FanPwm2FEnState/1  "sTmOut_D_u8FanPwm2FEnState"
  sTmDiag_D_u8BattCooltPmp2FEnState/1 -> Conversion39/1
  Conversion39/1 -> sTmOut_D_u8BattCooltPmp2FEnState/1  "sTmOut_D_u8BattCooltPmp2FEnState"
  sTmDiag_D_u8EmCooltPmp2FEnState/1 -> Conversion40/1
  Conversion40/1 -> sTmOut_D_u8EmCooltPmp2FEnState/1  "sTmOut_D_u8EmCooltPmp2FEnState"
  sTmDiag_D_u8PTCPumpSpd2FEnState/1 -> Conversion41/1
  Conversion41/1 -> sTmOut_D_u8PTCPumpSpd2FEnState/1  "sTmOut_D_u8PTCPumpSpd2FEnState"
  sTmDiag_D_u8EctvVlvMoveEna2FEnaState/1 -> Conversion42/1
  Conversion42/1 -> sTmOut_D_u8EctvVlvMoveEna2FEnaState/1  "sTmOut_D_u8EctvVlvMoveEna2FEnaState"
  sTmDiag_D_u8EctvVlvPos2FEnaState/1 -> Conversion43/1
  Conversion43/1 -> sTmOut_D_u8EctvVlvPos2FEnaState/1  "sTmOut_D_u8EctvVlvPos2FEnaState"
  sTmDiag_D_u8BctvVlvRef2FEnaState/1 -> Conversion44/1
  Conversion44/1 -> sTmOut_D_u8BctvVlvRef2FEnaState/1  "sTmOut_D_u8BctvVlvRef2FEnaState"
  sTmDiag_D_u8BctvVlvPos2FEnaState/1 -> Conversion45/1
  Conversion45/1 -> sTmOut_D_u8BctvVlvPos2FEnaState/1  "sTmOut_D_u8BctvVlvPos2FEnaState"
  sTmDiag_D_u8BcfvVlvRef2FEnaState/1 -> Conversion46/1
  Conversion46/1 -> sTmOut_D_u8BcfvVlvRef2FEnaState/1  "sTmOut_D_u8BcfvVlvRef2FEnaState"
  sTmDiag_D_u8BcfvVlvPos2FEnaState/1 -> Conversion47/1
  Conversion47/1 -> sTmOut_D_u8BcfvVlvPos2FEnaState/1  "sTmOut_D_u8BcfvVlvPos2FEnaState"
  sTmDiag_D_u8BexvCal2FEnaState/1 -> Conversion48/1
  Conversion48/1 -> sTmOut_D_u8BexvCal2FEnaState/1  "sTmOut_D_u8BexvCal2FEnaState"
  sTmDiag_D_u8BexvMoveEna2FEnaState/1 -> Conversion49/1
  Conversion49/1 -> sTmOut_D_u8BexvMoveEna2FEnaState/1  "sTmOut_D_u8BexvMoveEna2FEnaState"
  sTmDiag_D_u8BexvPosnReq2FEnaState/1 -> Conversion50/1
  Conversion50/1 -> sTmOut_D_u8BexvPosnReq2FEnaState/1  "sTmOut_D_u8BexvPosnReq2FEnaState"
  sTmDiag_D_u8CexvCal2FEnaState/1 -> Conversion51/1
  Conversion51/1 -> sTmOut_D_u8CexvCal2FEnaState/1  "sTmOut_D_u8CexvCal2FEnaState"
  sTmDiag_D_u8CexvMoveEna2FEnaState/1 -> Conversion52/1
  Conversion52/1 -> sTmOut_D_u8CexvMoveEna2FEnaState/1  "sTmOut_D_u8CexvMoveEna2FEnaState"
  sTmDiag_D_u8CexvPosnReq2FEnaState/1 -> Conversion53/1
  Conversion53/1 -> sTmOut_D_u8CexvPosnReq2FEnaState/1  "sTmOut_D_u8CexvPosnReq2FEnaState"
  sTmDiag_D_u8EexvCal2FEnaState/1 -> Conversion54/1
  Conversion54/1 -> sTmOut_D_u8EexvCal2FEnaState/1  "sTmOut_D_u8EexvCal2FEnaState"
